simulink model "QCar2_DetailedScenario-2025a"  (R2025a)
settings: Solver=ode2  StartTime=0.0  StopTime=inf  FixedStep=1/100  RelTol=1e-3  EnableMultiTasking=on
model workspace (MAT data in the model file):
  XY_OFFSET = Simulink.Parameter
  XY_OFFSET.Value = [0 0]
  XY_OFFSET.Complexity = 'real'
  XY_OFFSET.Dimensions = [1 2]
  XY_OFFSET.DataType = 'double'
  camera_rate = Simulink.Parameter
  camera_rate.Value = Simulink.data.Expression
  camera_rate.Value.ExpressionString = "qc_get_step_size * ceil(1/30 / qc_get_step_size)"
  camera_rate.Complexity = 'real'
  camera_rate.Dimensions = -1
  camera_rate.DataType = 'auto'
  depth_rate = Simulink.Parameter
  depth_rate.Value = Simulink.data.Expression
  depth_rate.Value.ExpressionString = "qc_get_step_size * ceil(1/30 / qc_get_step_size)"
  depth_rate.Complexity = 'real'
  depth_rate.Dimensions = -1
  depth_rate.DataType = 'auto'
  path_to_pickup = Simulink.Parameter
  path_to_pickup.Value = [-12.05  -8.3; -10.5  -9; -8  -10; -6  -10.5; -4  -10.8; -2  -10.9; 0  -10.95; 2  -10.95; 4  -10.9; 6  -10.85; 8  -10.85; 10  -10.9; 12  -10.92; 14  -10.92; 16  -10.5; 18  -9; 19.5  -7.5; 20.5  -5.5; 21  -4; 21.5  -3; 21.8  -1.5; 22  0; 22.1  2; 22.15  4; 22.15  6; 22.15  8; 22.15  10; 22.15  12; 22.15  14; 22.15  16; 22.15  18; 22.1  20; 22.1  22; 22.1  24; 22.1  26; 22.1  28; 22.05  30; 22  32; 21.9  34; 21.7  36; 21.4  38; 21  40; 20.5  41.5; 19.8  43; 18.8  44; 17.5  44.5; 16  44.8; 14  44.9; 12  44.92; 10  44.92; 8  44.92; 6  44.92; 4  44.92; 2  44.92; 1.25  44.5; 1.25  43.95]
  path_to_pickup.Complexity = 'real'
  path_to_pickup.Dimensions = [56 2]
  path_to_pickup.DataType = 'double'
  path_to_pickup_tight = Simulink.Parameter
  path_to_pickup_tight.Value = [-12.05  -8.3; -10.5  -9; -8  -10; -6  -10.5; -4  -10.8; -2  -10.9; 0  -10.95; 2  -10.95; 4  -10.9; 6  -10.85; 8  -10.85; 10  -10.9; 12  -10.92; 14  -10.92; 16  -10.5; 18  -9; 19.5  -7.5; 20.5  -5.5; 21  -4; 21.5  -3; 21.8  -1.5; 22  0; 22.1  2; 22.15  4; 22.15  6; 22.15  8; 22.15  10; 22.15  12; 22.15  14; 22.15  16; 22.15  18; 22.1  20; 22.1  22; 22.1  24; 22.1  26; 22.1  28; 22.05  30; 22  32; 21.9  34; 21.7  36; 21.4  38; 21  40; 20.5  41.5; 19.8  43; 18.8  44; 17.5  44.5; 16  44.8; 14  44.9; 12  44.92; 10  44.92; 8  44.92; 6  44.92; 4  44.92; 2  44.92; 1.25  44.5; 1.25  43.95]
  path_to_pickup_tight.Complexity = 'real'
  path_to_pickup_tight.Dimensions = [56 2]
  path_to_pickup_tight.DataType = 'double'
undefined symbols (not defined in the file or in its folder): gcbh, HIL, JPEG, Point, qc_get_step_size, Video3D, video_display_show
libraries: quarc_library x37, simulink x16
(part 1 of 3)
settings Model: SimulationMode=external  ExtModeTrigDuration=10000  Creator=User  LastModifiedBy=ricar
settings SolverCC: PositivePriorityOrder=on  AutoInsertRateTranBlk=on
settings DataIOCC: ReturnWorkspaceOutputs=off
settings DebuggingCC: AlgebraicLoopMsg=none  ParameterPrecisionLossMsg=none  UnconnectedInputMsg=warning  UnconnectedOutputMsg=warning  UnconnectedLineMsg=warning  ArithmeticOperatorsInVariantConditions=warning
settings ModelReferenceCC: EnableRefExpFcnMdlSchedulingChecks=on
settings SFSimCC: SimUseLocalCustomCode=off  CustomCodeUndefinedFunction=UseInterfaceOnly
settings RTWCC: RTWUseLocalCustomCode=off  Toolchain=QUARC win64 | nmake (64-bit Windows)  BuildConfiguration=Faster Runs  GPUComputeCapability=3.5

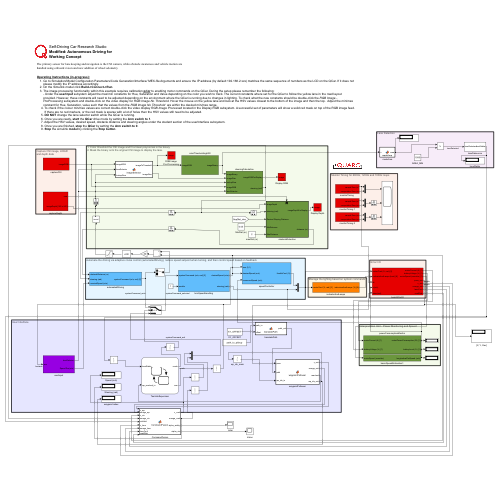
[thumbnail: Simulink's stored preview of the top-level diagram]
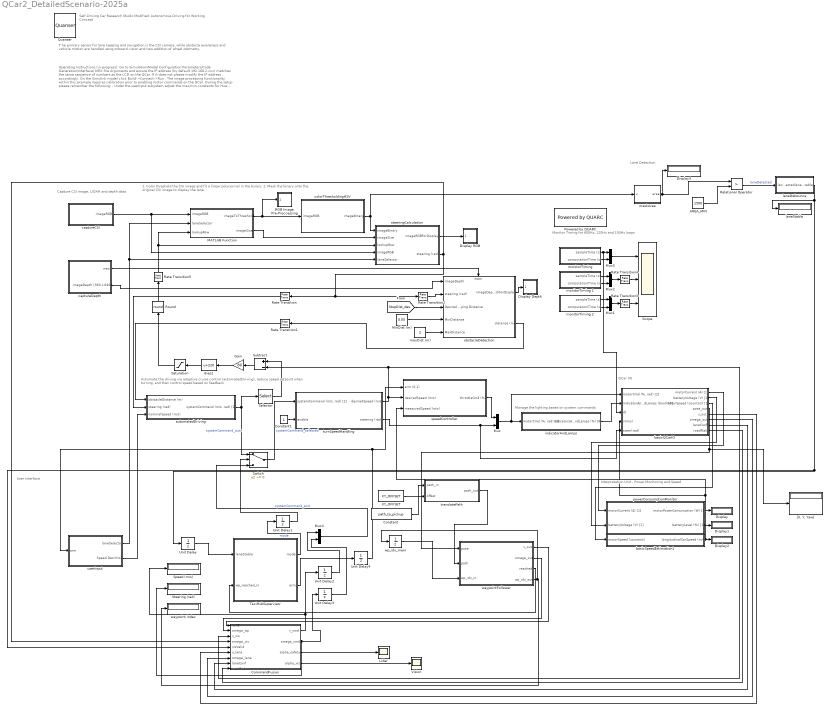
== system QCar2_DetailedScenario-2025a ==
  note: User Interface
  note: Operating Instructions (in-progress):
      | Go to Simulation/Model Configuration Parameters/Code Generation/Interface/ MEX-file Arguments and ensure the IP address (by default 192.168.2.xxx) matches the same sequence of numbers as the LCD on the QCar. If it does not please modify the IP address accordingly.
      | On the Simulink model click Build->Connect->Run .
      | The image processing functionality within this example requires calibration prior to enabling motor commands on the QCar. During the setup please remember the following:
      | - Under the userInput subystem adjust the max/min constants for Hue, Saturation and Value depending on the color you wish to track. The current constants where set for the QCar to follow the yellow lane in the road layout provided. However, these constants will need to be adjusted depending on the environment where the QCar is running due to changes in lighting. To check what the new constants should be double-click the RGB Image -PreProcessing subsystem and double-click on the video display for RGB Image No Threshold . Hover the mouse on the yellow lane and look at the HSV values closest to the bottom of the image and then the top. Adjust the min/max constant for Hue, Saturation, value such that the values from the RGB Image No Threshold are within the desired min/max range.
      | 4. To check if the colour min/max values are correct double-click the video display RGB Image Processed located in the Display RGB subsystem. A successful set of parameters will show a solid red mask on top of the RGB image feed.
      | If there are no red markers, or the red mask is sparse with a lot of holes then the HSV values still need to be adjusted.
      | 5. DO NOT change the lane selector switch while the QCar is running.
      | 6. Once you are ready, start the QCar drive mode by setting the Arm switch to 1 .
      | 7. Adjust the HSV values, desired speed, obstacle distance and steering angles under the student section of the userInterface subsystem.
      | 8. Once you are finished, stop the QCar by setting the Arm switch to 0 .
      | 9. Stop the simulink model by clicking the Stop button .
  note: Monitor Timing for 600Hz, 120Hz and 100Hz loops
  note: Manage the lighting based on system commands
  note: QCar I/O
  note: Automate the driving via adaptive cruise control (automatedDriving), reduce speed setpoint when turning, and then control speed based on feedback
  note: Self-Driving Car Research Studio
      | Modified: Autonomous Driving for Working Concept
  note: Capture CSI image, LIDAR
      | and depth data
  note: 1. Color threshold the CSI image and fit a linear polynomial in the binary.
      | 2. Mask the binary onto the original CSI image to display the lane.
  note: T he primary sensor for lane keeping and navigation is the CSI camera, while obstacle awareness and vehicle motion are handled using onboard vision and new addition of wheel odometry.
  note: Interpretation Unit - Power Monitoring and Speed
  note: Lane Detection
  AREA_MIN : Constant  Value=1500
  Bias1 : Bias  Bias=220  SaturateOnIntegerOverflow=off
  CommandFusion : MATLAB Function  TreatAsAtomicUnit=on
  Constant : Constant  Value=path_to_pickup
  Constant1 : Constant
  Display{,1..3} (4 alike) : Display
      Display settings: Decimation=0.5/qc_get_step_size
      Display1 settings: Decimation=0.5/qc_get_step_size
      Display2 settings: Decimation=0.5/qc_get_step_size
  Display Depth : Subsystem
  Display RGB : Subsystem
  Gain : Gain  Gain=80
  Lidar : Scope
      settings: ActiveDisplayYMinimum=0.063200000000000034  ActiveDisplayYMaximum=0.26320000000000005  DataLoggingVariableName=ScopeData6
  MATLAB Function : MATLAB Function  TreatAsAtomicUnit=on
  MinDist (m) : Constant  Value=0.05
  Mux{,1..4} (5 alike) : Mux  Inputs=2
  Powered by QUARC : quarc_library/Logos/Powered by QUARC
  Quanser : quarc_library/Logos/Quanser
  RGB Image Pre-Proccessing : Subsystem
  Rate Transition{,1,3..5} (5 alike) : RateTransition
  Rate Transition2 : RateTransition  Deterministic=off
  Relational Operator : RelationalOperator  Operator=>  OutDataTypeStr=boolean  RndMeth=Simplest  InputSameDT=off
  Round : Rounding  Operator=round
  Saturation : Saturate  UpperLimit=300  LowerLimit=220
  Scope : Scope  NumInputPorts=3
      settings: TimeSpan=60  Title=Timing: 500 Hz loop  ActiveDisplayYMinimum=-0.00084  ActiveDisplayYMaximum=0.00516  YLabel=s
  Selector : Selector  InputPortWidth=2  IndexOptions=Index vector (dialog)  Indices=[1]  OutputSizes=1
  Speed (m/s) : Display
  Steering (rad) : Display
  Subtract : Sum  Inputs=+-
  Switch : Switch  Criteria=u2 ~= 0  SaturateOnIntegerOverflow=off  InputSameDT=off
  "TaxiHubSupervisor " : Stateflow chart  TreatAsAtomicUnit=on
  Unit Delay{,1..4} (5 alike) : UnitDelay  SampleTime=-1  HasFrameUpgradeWarning=on
  Vision : Scope
      settings: ActiveDisplayYMinimum=-1  ActiveDisplayYMaximum=1  DataLoggingVariableName=ScopeData7
  XY_OFFSET : Constant  Value=XY_OFFSET
  "[X, Y, Yaw]" : Display
  automatedDriving : Subsystem
  basicQCarIO : Subsystem
  basicSpeedEstimation1 : Subsystem
  captureCSI : Subsystem
  captureDepth : Subsystem
  colorThresholdingHSV : Subsystem
  indicatorAndLamps : Subsystem
  laneDebounce : Subsystem
  laneStable : Display
  maskArea : MATLAB Function  TreatAsAtomicUnit=on
  maxDist (m) : Constant  Value=2
  "monitorTiming " : Subsystem
  monitorTiming 1 : Subsystem
  monitorTiming 2 : Subsystem
  obstacleDetection : Subsystem
  powerConsumptionMonitor : Subsystem
  speedController : Subsystem
  steeringCalculation : Subsystem
  translatePath : MATLAB Function  TreatAsAtomicUnit=on
  turnSpeedHandling : Subsystem
  userInput : Subsystem
  waypoint index : Display
  waypointFollower : MATLAB Function  TreatAsAtomicUnit=on
  wp_idx_mem : UnitDelay  InitialCondition=1  SampleTime=-1  HasFrameUpgradeWarning=on
  wires:
  Mux/1 -> basicQCarIO/1("motorCmd (%, rad) [2]"), indicatorAndLamps/1("motorCmd (%, rad) [2]")
  turnSpeedHandling/2(steering (rad)) -> basicQCarIO/5(steer(rad)), Mux/2
  Constant1/1 -> turnSpeedHandling/2(enable)
  indicatorAndLamps/1(indicatorsAndLamps (%) [8]) -> basicQCarIO/2(indicatorAndLamps (bool) [8])
  captureDepth/2(imageDepth [360 x 640]) -> obstacleDetection/1(imageDepth)
  obstacleDetection/2(distance (m)) -> Rate Transition1/1
  speedController/1(throttleCmd (%)) -> Mux/1
  Rate Transition/1 -> automatedDriving/2(steering (rad))
  Rate Transition1/1 -> automatedDriving/1(obstacleDistance (m))
  Rate Transition2/1 -> obstacleDetection/2(steering (rad))
  obstacleDetection/1(imageDepthForDisplay) -> Display Depth/1(Image)
  captureCSI/1(imageRGB) -> steeringCalculation/4(imageRGB), MATLAB Function/1(imageRGB)
  monitorTiming 2/2(computationTime (s)) -> Mux1/2
  monitorTiming 2/1(sampleTime (s)) -> Mux1/1
  monitorTiming 1/2(computationTime (s)) -> Mux2/2
  monitorTiming 1/1(sampleTime (s)) -> Mux2/1
  "monitorTiming "/2(computationTime (s)) -> Mux3/2
  "monitorTiming "/1(sampleTime (s)) -> basicQCarIO/3(dt), Mux3/1
  Mux2/1 -> Rate Transition4/1
  Mux1/1 -> Rate Transition3/1
  Mux3/1 -> Scope/1
  Rate Transition3/1 -> Scope/3
  Rate Transition4/1 -> Scope/2
  captureDepth/1(new) -> obstacleDetection/Enable
  steeringCalculation/2(steering (rad)) -> CommandFusion/4(omega_vis), Rate Transition2/1, Rate Transition/1
  colorThresholdingHSV/1(imageBinary) -> maskArea/1(u), steeringCalculation/1(imageBinary)
  steeringCalculation/1(imageRGBForDisplay) -> Display RGB/1(Image)
  MATLAB Function/1(imageToThreshold) -> RGB Image Pre-Proccessing/1(Image), colorThresholdingHSV/1(imageRGB)
  MATLAB Function/2(imageSize) -> steeringCalculation/2(imageSize)
  turnSpeedHandling/1(desiredSpeed (m/s)) -> speedController/2(desiredSpeed (m/s)), CommandFusion/3(v_vis), Subtract/2
  Gain/1 -> Bias1/1
  Saturation/1 -> Round/1
  Selector/1 -> Subtract/1
  Subtract/1 -> Gain/1
  Bias1/1 -> Saturation/1
  Rate Transition5/1 -> steeringCalculation/3(lookupRow), MATLAB Function/3(lookupRow)
  userInput/1(laneSelector) -> steeringCalculation/5(laneSelector), MATLAB Function/2(laneSelector)
  userInput/2(Speed Des(m/s)) -> automatedDriving/3(nominalSpeed (m/s))
  [StopDist_des] -> obstacleDetection/3(Desired Stoping Distance)
  maxDist (m)/1 -> obstacleDetection/5(MaxDistance)
  MinDist (m)/1 -> obstacleDetection/4(MinDistance)
  Round/1 -> Rate Transition5/1
  basicQCarIO/1(motorCurrent (A) [1]) -> powerConsumptionMonitor/1(motorCurrent (A) [1])
  basicQCarIO/2(batteryVoltage (V) [1]) -> powerConsumptionMonitor/2(batteryVoltage (V) [1])
  basicQCarIO/3(motorSpeed (counts/s) [1]) -> basicSpeedEstimation1/1(motorSpeed (counts/s))
  powerConsumptionMonitor/1(motorPowerConsumption (W) [1]) -> Display/1
  basicSpeedEstimation1/1(longitudinalCarSpeed (m/s)) -> basicQCarIO/4(v(m/s)), speedController/3(measuredSpeed (m/s)), Display2/1
  powerConsumptionMonitor/2(batteryLevel (%) [1]) -> Display1/1
  automatedDriving/1("systemCommand (m/s, rad) [2]") -> Selector/1, Switch/1  "systemCommand_auto"
  Mux4/1 -> Switch/3  "systemCommand_exit"
  Switch/1 -> turnSpeedHandling/1("systemCommand (m/s, rad) [2]")  "systemCommand_selected"
  maskArea/1(area) -> Display3/1, Relational Operator/1
  AREA_MIN/1 -> Relational Operator/2
  Relational Operator/1 -> laneDebounce/1(laneDetected)  "laneDetected"
  laneDebounce/1(laneStable) -> CommandFusion/5(visValid), Unit Delay/1, laneStable/1
  Unit Delay/1 -> "TaxiHubSupervisor "/1(laneStable)
  wp_idx_mem/1 -> waypointFollower/3(wp_idx_in)
  waypointFollower/4(wp_idx_out) -> waypoint index/1, wp_idx_mem/1
  waypointFollower/3(reached) -> "TaxiHubSupervisor "/2(wp_reached_in)
  "TaxiHubSupervisor "/1(mode) -> Unit Delay1/1  "mode"
  Unit Delay1/1 -> Switch/2
  Unit Delay2/1 -> Mux4/1
  "TaxiHubSupervisor "/2(arm) -> Unit Delay4/1
  Unit Delay4/1 -> userInput/1(arm), speedController/1(arm (0,1))
  Unit Delay3/1 -> Mux4/2
  XY_OFFSET/1 -> translatePath/2(offset)
  Constant/1 -> translatePath/1(path_in)
  translatePath/1(path_out) -> waypointFollower/2(path)
  basicQCarIO/4(pose_out) -> "[X, Y, Yaw]"/1, waypointFollower/1(pose)
  basicQCarIO/5(v_out) -> CommandFusion/6(v_lane)
  basicQCarIO/6(omega_out) -> CommandFusion/7(omega_lane)
  waypointFollower/1(v_out) -> CommandFusion/1(v_wp)
  CommandFusion/1(v_cmd) -> Speed (m/s)/1, Unit Delay2/1
  basicQCarIO/7(laneConf) -> CommandFusion/8(laneConf)
  basicQCarIO/8(roadRisk) -> CommandFusion/9(roadRisk)
  CommandFusion/3(alpha_safety) -> Lidar/1
  waypointFollower/2(omega_out) -> CommandFusion/2(omega_wp)
  CommandFusion/4(alpha_vis) -> Vision/1
  CommandFusion/2(omega_cmd) -> Steering (rad)/1, Unit Delay3/1

== system QCar2_DetailedScenario-2025a/Display Depth ==
  Image : Inport
  Channel : quarc_library/Signal Routing/Channel  channel=0  buffer_size=1
  Video Display : quarc_library/Multimedia/Video Display  Tag=QCar2_DetailedScenario/Display Depth/Video Display  sample_time=-1  use_hardware=on
  wires:
  Image/1 -> Channel/1
  Channel/1 -> Video Display/1

== system QCar2_DetailedScenario-2025a/Display RGB ==
  Image : Inport
  Channel : quarc_library/Signal Routing/Channel  channel=1  buffer_size=1
  Video Display : quarc_library/Multimedia/Video Display  Tag=QCar2_DetailedScenario/Display RGB/Video Display  sample_time=-1  use_hardware=on
  wires:
  Image/1 -> Channel/1
  Channel/1 -> Video Display/1

== system QCar2_DetailedScenario-2025a/RGB Image Pre-Proccessing ==
  Image : Inport
  Channel : quarc_library/Signal Routing/Channel  channel=2  buffer_size=1
  Video Display : quarc_library/Multimedia/Video Display  Tag="QCar2_DetailedScenario/RGB Image  Pre-Proccessing/Video Display"  sample_time=-1  use_hardware=on
  wires:
  Image/1 -> Channel/1
  Channel/1 -> Video Display/1

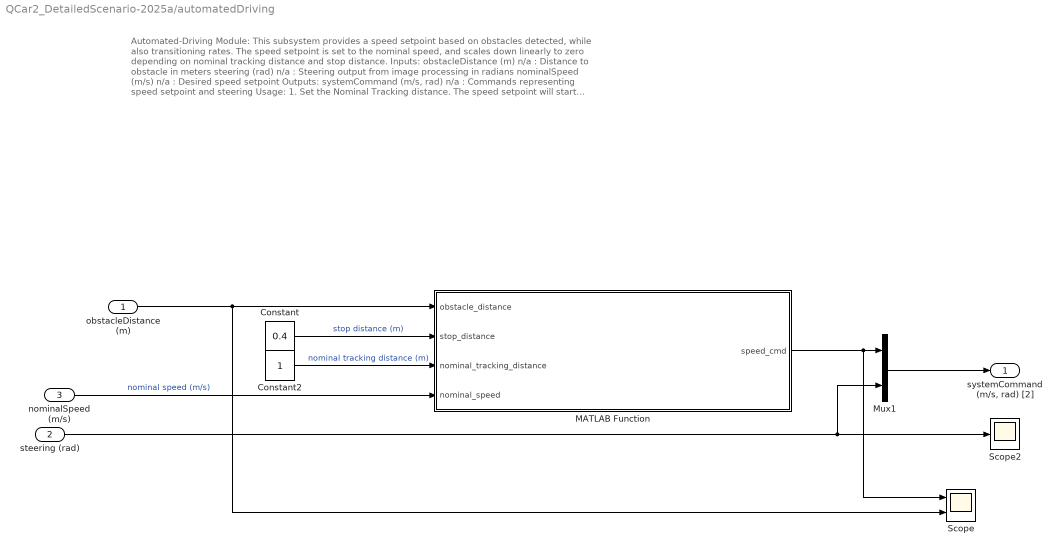
== system QCar2_DetailedScenario-2025a/automatedDriving ==
  note: Automated-Driving Module:
      |
      | This subsystem provides a speed setpoint based on obstacles detected, while also transitioning rates. The speed setpoint is set to the nominal speed, and scales down linearly to zero depending on nominal tracking distance and stop distance.
      |
      | Inputs:
      | obstacleDistance (m) n/a : Distance to obstacle in meters
      | steering (rad) n/a : Steering output from image processing in radians
      | nominalSpeed (m/s) n/a : Desired speed setpoint
      |
      | Outputs:
      | systemCommand (m/s, rad) n/a : Commands representing speed setpoint and steering
      |
      | Usage:
      | 1. Set the Nominal Tracking distance. The speed setpoint will start decreasing if the obstacle distance is less than this threshold.
      | 2. Set the Stop Distance. The speed setpoint will scale down to 0 when the the obstacle distance reaches this threshold.
  obstacleDistance (m) : Inport
  steering (rad) : Inport  Port=2
  nominalSpeed (m/s) : Inport  Port=3
  Constant : Constant  Value=0.4
  Constant2 : Constant
  MATLAB Function : MATLAB Function  TreatAsAtomicUnit=on
  Mux1 : Mux  Inputs=2
  Scope : Scope  NumInputPorts=2
      settings: ActiveDisplayYMinimum=-0.06597  ActiveDisplayYMaximum=1.21757
  Scope2 : Scope
      settings: ActiveDisplayYMinimum=-0.625  ActiveDisplayYMaximum=0.625  DataLoggingVariableName=ScopeData2
  "systemCommand (m/s, rad) [2]" : Outport  VectorParamsAs1DForOutWhenUnconnected=off
  wires:
  nominalSpeed (m/s)/1 -> MATLAB Function/4(nominal_speed)  "nominal speed (m/s)"
  Constant2/1 -> MATLAB Function/3(nominal_tracking_distance)  "nominal tracking distance (m)"
  Constant/1 -> MATLAB Function/2(stop_distance)  "stop distance (m)"
  MATLAB Function/1(speed_cmd) -> Scope/1, Mux1/1
  steering (rad)/1 -> Mux1/2, Scope2/1
  Mux1/1 -> "systemCommand (m/s, rad) [2]"/1
  obstacleDistance (m)/1 -> Scope/2, MATLAB Function/1(obstacle_distance)

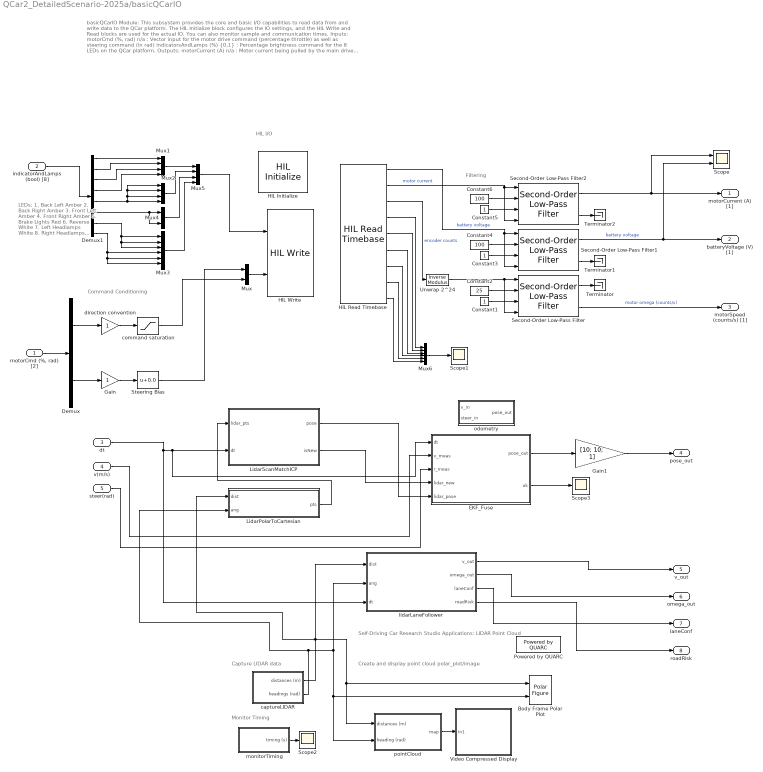
== system QCar2_DetailedScenario-2025a/basicQCarIO ==
  note: Filtering
  note: basicQCarIO Module:
      |
      | This subsystem provides the core and basic I/O capabilities to read data from and write data to the QCar platform. The HIL Initialize block configures the IO settings, and the HIL Write and Read blocks are used for the actual IO. You can also monitor sample and communication times.
      |
      | Inputs:
      | motorCmd (%, rad) n/a : Vector input for the motor drive command (percentage throttle) as well as steering command (in rad)
      | indicatorsAndLamps (%) {0,1} : Percentage brightness command for the 8 LEDs on the QCar platform.
      |
      | Outputs:
      | motorCurrent (A) n/a : Motor current being pulled by the main drive motor
      | batteryVoltage (V) {0, 12.6} : Current battery voltage reading
      | motorSpeed (counts/s) n/a : Drive motor speed measured using an encoder (do not confuse with wheel speed as this measurement is at the drive shaft)
  note: HIL I/O
  note: Command Conditioning
  note: LEDs:
      | 1. Back Left Amber
      | 2. Back Right Amber
      | 3. Front Left Amber
      | 4. Front Right Amber
      | 5. Brake Lights Red
      | 6. Reverse White
      | 7. Left Headlamps White
      | 8. Right Headlamps White
  note: Create and display point cloud polar_plot/image
  note: Self-Driving Car Research Studio
      | Applications: LIDAR Point Cloud
  note: Capture LIDAR data
  note: Monitor Timing
  "motorCmd (%, rad) [2]" : Inport
  indicatorAndLamps (bool) [8] : Inport  Port=2
  dt : Inport  Port=3
  v(m/s) : Inport  Port=4
  steer(rad) : Inport  Port=5
  Body Frame Polar Plot : quarc_library/Sinks/Figures/Polar Figure  figure_mode=Use figure window  figure_tag=figure1  axes_tag=axes1  plot_mode=Frame-based  minimum_rho=0  maximum_rho=5  minimum_theta=0  maximum_theta=360  zero_location=top  direction=counterclockwise  buffer_size=1000  update_rate=1  sample_time=-1  initial_position="898  139  994  602"  initial_visibility=off  line1_style=None  line1_width=0.5  line1_color=[0 0.4470 0.7410]  marker1=Point (.)  marker1_size=1  marker1_edge_color=[0 0.447059 0.741176]  marker1_face_color=[0 0.447059 0.741176]  line2_style=Solid line (-)  line2_width=0.5  line2_color=[0.85098 0.32549 0.0980392]  marker2=None  marker2_size=6  marker2_edge_color=[0.85098 0.32549 0.0980392]  marker2_face_color=[0.85098 0.32549 0.0980392]  line3_style=Solid line (-)  line3_width=0.5  line3_color=[0.929412 0.694118 0.12549]  marker3=None  marker3_size=6  marker3_edge_color=[0.929412 0.694118 0.12549]  marker3_face_color=[0.929412 0.694118 0.12549]  line4_style=Solid line (-)  line4_width=0.5  line4_color=[0.494118 0.184314 0.556863]  marker4=None  marker4_size=6  marker4_edge_color=[0.494118 0.184314 0.556863]  marker4_face_color=[0.494118 0.184314 0.556863]  line5_style=Solid line (-)  line5_width=0.5  line5_color=[0.466667 0.67451 0.188235]  marker5=None  marker5_size=6  marker5_edge_color=[0.466667 0.67451 0.188235]  marker5_face_color=[0.466667 0.67451 0.188235]
      settings: SourceProductName=QUARC Targets
  Constant1 : Constant
  Constant2 : Constant  Value=25
  Constant3 : Constant
  Constant4 : Constant  Value=100
  Constant5 : Constant
  Constant6 : Constant  Value=100
  Demux : Demux  Outputs=2
  Demux1 : Demux  Outputs=8
  EKF_Fuse : MATLAB Function  TreatAsAtomicUnit=on
  Gain : Gain
  Gain1 : Gain  Gain=[10; 10; 1]
  HIL Initialize : quarc_library/Data Acquisition/Generic/Configuration/HIL Initialize  object_name=HIL-1  board_type=qcar2  board_number=0@tcpip://localhost:18960  board_options=gyro_fs=250;gyro_rate=500;gyro_bw=125;gyro_ord=3;accel_fs=16;accel_rate=1000;accel_bw=250;accel_ord=3;temp_bw=4000;enc0_dir=0;enc1_dir=0;enc2_dir=0;steer_bias=0.05;  exclusive=off  active=on  hardware_clocks=[]  clock_modes=[]  initial_clock_frequencies=[]  set_clock_params_at_start=off  set_clock_params_at_switch_in=off  set_clock_frequencies_at_start=off  set_clock_frequencies_at_switch_in=off  analog_input_channels=[0:4]  analog_input_configurations=[]  analog_input_maximums=[3.3]  analog_input_minimums=[0]  set_analog_input_params_at_start=off  set_analog_input_params_at_switch_in=off  analog_output_channels=[]  analog_output_maximums=[]  analog_output_minimums=[]  initial_analog_outputs=[]  final_analog_outputs=[]  watchdog_analog_outputs=[]  set_analog_output_params_at_start=off  set_analog_output_params_at_switch_in=off  set_analog_outputs_at_start=off  set_analog_outputs_at_switch_in=off  set_analog_outputs_at_terminate=off  set_analog_outputs_at_switch_out=off  set_analog_outputs_on_watchdog=off  digital_input_channels=[0:14]  digital_output_channels=[11:26]  digital_output_configuration=[]  initial_digital_outputs=[0]  final_digital_outputs=[0]  watchdog_digital_outputs=[0]  set_digital_output_params_at_start=off  set_digital_output_params_at_switch_in=off  set_digital_outputs_at_start=on  set_digital_outputs_at_switch_in=off  set_digital_outputs_at_terminate=on  set_digital_outputs_at_switch_out=off  set_digital_outputs_on_watchdog=off  encoder_channels=[0:2]  quadrature=[4]  encoder_filter_frequency=100e6/1  initial_encoder_counts=[0]  set_encoder_params_at_start=on  set_encoder_params_at_switch_in=off  set_encoder_counts_at_start=on  set_encoder_counts_at_switch_in=off  pwm_channels=[0:1]  pwm_modes=[0]  pwm_frequency=180e6/4096  pwm_configuration=[0]  pwm_alignment=[0]  pwm_polarity=[1]  pwm_leading_deadband=[]  pwm_trailing_deadband=[]  initial_pwm_outputs=[0]  final_pwm_outputs=[0]  watchdog_pwm_outputs=[0]  set_pwm_params_at_start=on  set_pwm_params_at_switch_in=off  set_pwm_outputs_at_start=on  set_pwm_outputs_at_switch_in=off  set_pwm_outputs_at_terminate=on  set_pwm_outputs_at_switch_out=off  set_pwm_outputs_on_watchdog=off  other_output_channels=[1000 11000]  initial_other_outputs=[0]  final_other_outputs=[0]  watchdog_other_outputs=[0]  set_other_outputs_at_start=on  set_other_outputs_at_switch_in=off  set_other_outputs_at_terminate=on  set_other_outputs_at_switch_out=off  set_other_outputs_on_watchdog=off
  HIL Read Timebase : quarc_library/Data Acquisition/Generic/Timebases/HIL Read Timebase  object_name=HIL-1  clock=0  analog_channels=[2 4]  encoder_channels=[0]  digital_channels=[]  other_channels=[3000:3002 4000:4002]  active=on  vector_output=off  data_type_mode=Inherit via back propagation  encoder_data_type=double  digital_data_type=boolean  overflow_mode=Synchronize (for simulated cards only)  samples_in_buffer=max(ceil(1/qc_get_step_size), 1)*0+1
  HIL Write : quarc_library/Data Acquisition/Generic/Immediate I//O/HIL Write  object_name=HIL-1  analog_channels=[]  pwm_channels=[]  digital_channels=[17:18 25:26 11:16 19:24]  other_channels=[1000 11000]  sample_time=qc_get_step_size  active=on  vector_input=on
  LidarPolarToCartesian : MATLAB Function  TreatAsAtomicUnit=on
  LidarScanMatchICP : MATLAB Function  TreatAsAtomicUnit=on
  Mux : Mux  Inputs=2
  Mux1 : Mux
  Mux2 : Mux
  Mux3 : Mux  Inputs=6
  Mux4 : Mux  Inputs=2
  Mux5 : Mux
  Mux6 : Mux  Inputs=6
  Powered by QUARC : quarc_library/Logos/Powered by QUARC
  Scope : Scope  NumInputPorts=2
      settings: ActiveDisplayYMinimum=-1.03564  ActiveDisplayYMaximum=12.37845  DataLoggingVariableName=ScopeData4
  Scope1 : Scope
  Scope2 : Scope
      settings: ActiveDisplayYMinimum=-0.0098  ActiveDisplayYMaximum=0.1122
  Scope3 : Scope
      settings: ActiveDisplayYMinimum=-1  ActiveDisplayYMaximum=1  DataLoggingVariableName=ScopeData5
  Second-Order Low-Pass Filter : quarc_library/Continuous/Second-Order Low-Pass Filter  params_source=External (input ports)  input_width=1  input_zeta=1  input_init=0
  Second-Order Low-Pass Filter1 : quarc_library/Continuous/Second-Order Low-Pass Filter  params_source=External (input ports)  input_width=1  input_zeta=1  input_init=0
  Second-Order Low-Pass Filter2 : quarc_library/Continuous/Second-Order Low-Pass Filter  params_source=External (input ports)  input_width=1  input_zeta=1  input_init=0
  Steering Bias : Bias  Bias=0.0  SaturateOnIntegerOverflow=off
  Terminator : Terminator
  Terminator1 : Terminator
  Terminator2 : Terminator
  Unwrap 2^24 : quarc_library/Discontinuities/Inverse Modulus  modulus=16777215  output_derivative=off  output_revolutions=off  max_x=Inf  min_x=-Inf
  Video Compressed Display : Subsystem  LoadFcn=set_param(gcbh, 'UserData', gcb);  StartFcn=video_display_show([gcb, '/Video Display'], 'add', gcb);  mask(Video Compressed Display){algorithm=JPEG, quality=50, sample_time=-1, use_hardware=on}
      mask prompts: algorithm "Compression algorithm:"; quality "Compression quality (0-100):"; sample_time "Sample time (seconds):"; use_hardware "Use hardware acceleration for video display"
      mask help: Displays a video stream on the host, using compression to minimize bandwidth.
      mask init:
      | qc_set_display('Video\nCompressed\nDisplay');
      settings: UndoDeleteFcn=set_param(gcbh, 'UserData', gcb);  OpenFcn=video_display_show([gcb, '/Video Display'], 'show', gcb);  PreDeleteFcn=video_display_show([gcb, '/Video Display'], 'delete');
      settings: CopyFcn=|
      | set_param(gcbh, 'UserData', gcb);
      | set_param(gcbh, 'LinkStatus', 'none');
      settings: NameChangeFcn=|
      | video_display_show([get_param(gcbh, 'UserData'), '/Video Display'], 'rename', [gcb, '/Video Display']);
      | video_display_show([gcb, '/Video Display'], 'add', gcb);
      | set_param(gcbh, 'UserData', gcb);
      mask Help: web(qc_get_block_help_path(gcb));
      mask TypeOptions algorithm: Image Compress/algorithm
      mask TypeOptions quality: Image Compress/quality
      mask TypeOptions sample_time: Video Display/sample_time
      mask TypeOptions use_hardware: Video Display/use_hardware
      mask Display:
      | patch([0.98591 0.98591 0.62618 0.59072 0.56147   0.536   0.536  0.5441 0.56912 0.59207 0.60881 0.62276 0.63527 0.64364  0.6485  0.6485 0.64706 0.64499 0.63662 0.62411 0.61232 0.59837 0.58307 0.56147   0.536   0.536  0.5441  0.5747 0.60953 0.63662 0.67001  0.7034 0.72851 0.75425 0.77927 0.80294 0.82454 0.84119 0.85865 0.87395 0.88574 0.89339  0.8969 0.89969 0.89969 0.89267  0.8816 0.87044 0.85649  0.8384 0.81824 0.80294 0.78764 0.77513 0.76676 0.75776 0.76397 0.77513 0.79178 0.80987 0.82796 0.84326 0.86207 0.98528],[0.18689 0.05522 0.05522 0.05171 0.05171    0.05 0.18338 0.18338 0.19148 0.20435 0.22298 0.24863 0.28589 0.33125 0.38138 0.55139 0.59801 0.63761 0.68189 0.72149 0.74939 0.76694 0.77855 0.79367 0.79952 0.92768 0.92768 0.92768 0.92417 0.92066 0.91364  0.9032 0.89384 0.88106 0.86594 0.85073 0.82634 0.80537 0.77855 0.74363 0.70403 0.65858 0.61079 0.59099 0.41513 0.37202 0.31847 0.29048 0.25556 0.23342  0.2102 0.19382 0.18221 0.17285 0.16943 0.16124  0.1589 0.16241 0.16709 0.17168  0.1787 0.18221 0.18689 0.18689],[0.9,0.90,0.91])
      | patch([0.536 0.52601 0.46823 0.44528 0.41603 0.39101 0.35555 0.33116 0.31451 0.29291  0.2804 0.26717 0.25322 0.23999 0.22406 0.20732 0.19337 0.17528 0.15935 0.14396 0.13217 0.11759 0.10922 0.10085 0.09671 0.09392 0.09041 0.08906 0.08906 0.09464  0.0995 0.10778 0.11894 0.13145 0.14675 0.16349 0.17672 0.19409 0.20732 0.22406 0.23999 0.26159 0.27833 0.29849 0.31793 0.33602 0.35411 0.37085 0.39245 0.41603   0.536   0.536 0.53159 0.46409   0.446 0.42026 0.39587 0.37571 0.36113 0.34925 0.34088 0.33809 0.33809 0.34088 0.34583 0.35627 0.36392 0.38129 0.39587 0.41117 0.42719 0.44672  0.4676 0.48353 0.48353 0.52394   0.536],[0.05 0.04829 0.04712 0.04712 0.04829 0.05063 0.05405 0.05873 0.06107 0.06692 0.07043 0.07619 0.08087 0.08672 0.09482 0.10652 0.11696 0.13325  0.1508 0.17168 0.19499 0.22415 0.25439 0.28472 0.31379 0.35456 0.38489 0.41513 0.58055 0.63878 0.68774 0.72149 0.75641 0.78089 0.80537 0.82859 0.84029 0.85658 0.86594 0.87404  0.8834 0.89267 0.90086 0.90788 0.91247 0.91832 0.92066   0.923 0.92651 0.92768 0.92768 0.79952 0.79952 0.79952 0.79718 0.78899 0.77153 0.75056 0.72149 0.68072 0.62249  0.5549 0.41396 0.37085 0.33242 0.28121 0.25205 0.22181 0.20552 0.19499 0.18572 0.18221 0.17753 0.17636 0.17753  0.1787  0.1787],[0.9,0.90,0.91])
      | disp('Video\nCompressed\nDisplay');
  captureLIDAR : Subsystem
  command saturation : Saturate  UpperLimit=0.20  LowerLimit=-0.20
  direction convention : Gain
  lidarLaneFollower : MATLAB Function  TreatAsAtomicUnit=on
  "monitorTiming " : Subsystem
  odometry : Subsystem
  pointCloud : Subsystem
  motorCurrent (A) [1] : Outport  VectorParamsAs1DForOutWhenUnconnected=off
  batteryVoltage (V) [1] : Outport  Port=2  VectorParamsAs1DForOutWhenUnconnected=off
  motorSpeed (counts/s) [1] : Outport  Port=3  VectorParamsAs1DForOutWhenUnconnected=off
  pose_out : Outport  Port=4
  v_out : Outport  Port=5  OutDataTypeStr=double  PortDimensions=1
  omega_out : Outport  Port=6  OutDataTypeStr=double  PortDimensions=1
  laneConf : Outport  Port=7
  roadRisk : Outport  Port=8
  wires:
  Second-Order Low-Pass Filter2/1 -> Scope/1, motorCurrent (A) [1]/1
  Constant2/1 -> Second-Order Low-Pass Filter/2
  Unwrap 2^24/1 -> Second-Order Low-Pass Filter/1, Second-Order Low-Pass Filter/4
  Second-Order Low-Pass Filter/1 -> Terminator/1
  Constant3/1 -> Second-Order Low-Pass Filter1/3
  Second-Order Low-Pass Filter1/1 -> Scope/2, batteryVoltage (V) [1]/1  "battery voltage"
  Constant5/1 -> Second-Order Low-Pass Filter2/3
  Second-Order Low-Pass Filter1/2 -> Terminator1/1
  HIL Read Timebase/1 -> Second-Order Low-Pass Filter1/4, Second-Order Low-Pass Filter1/1  "battery voltage"
  Constant6/1 -> Second-Order Low-Pass Filter2/2
  Second-Order Low-Pass Filter/2 -> motorSpeed (counts/s) [1]/1  "motor omega (counts/s)"
  Second-Order Low-Pass Filter2/2 -> Terminator2/1
  Constant4/1 -> Second-Order Low-Pass Filter1/2
  Constant1/1 -> Second-Order Low-Pass Filter/3
  HIL Read Timebase/3 -> Unwrap 2^24/1  "encoder counts"
  HIL Read Timebase/2 -> Second-Order Low-Pass Filter2/1, Second-Order Low-Pass Filter2/4  "motor current"
  Mux5/1 -> HIL Write/1
  "motorCmd (%, rad) [2]"/1 -> Demux/1
  Mux3/1 -> Mux5/4
  Demux1/4 -> Mux1/4
  Demux1/3 -> Mux1/3
  Demux1/6 -> Mux4/2, Mux4/1
  Steering Bias/1 -> Mux/1
  Demux1/8 -> Mux3/5, Mux3/6, Mux3/4
  Mux1/1 -> Mux5/1
  Demux1/7 -> Mux3/2, Mux3/3, Mux3/1
  Demux/1 -> direction convention/1
  Demux1/5 -> Mux2/4, Mux2/3, Mux2/2, Mux2/1
  Mux2/1 -> Mux5/2
  Mux/1 -> HIL Write/2
  indicatorAndLamps (bool) [8]/1 -> Demux1/1
  Demux/2 -> Gain/1
  Mux4/1 -> Mux5/3
  command saturation/1 -> Mux/2
  Demux1/2 -> Mux1/2
  direction convention/1 -> command saturation/1
  Gain/1 -> Steering Bias/1
  Demux1/1 -> Mux1/1
  Mux6/1 -> Scope1/1
  HIL Read Timebase/9 -> Mux6/6
  HIL Read Timebase/7 -> Mux6/4
  HIL Read Timebase/5 -> Mux6/2
  HIL Read Timebase/8 -> Mux6/5
  HIL Read Timebase/6 -> Mux6/3
  HIL Read Timebase/4 -> Mux6/1
  "monitorTiming "/1(timing (s)) -> Scope2/1
  captureLIDAR/2(headings (rad)) -> LidarPolarToCartesian/2(ang), lidarLaneFollower/2(ang), Body Frame Polar Plot/2, pointCloud/2(heading (rad))
  pointCloud/1(map) -> Video Compressed Display/1(In1)
  captureLIDAR/1(distances (m)) -> lidarLaneFollower/1(dist), LidarPolarToCartesian/1(dist), pointCloud/1(distances (m)), Body Frame Polar Plot/1
  LidarPolarToCartesian/1(pts) -> LidarScanMatchICP/1(lidar_pts)
  LidarScanMatchICP/1(pose) -> EKF_Fuse/5(lidar_pose)
  LidarScanMatchICP/2(isNew) -> EKF_Fuse/4(lidar_new)
  dt/1 -> lidarLaneFollower/3(dt), EKF_Fuse/1(dt), LidarScanMatchICP/2(dt)
  v(m/s)/1 -> EKF_Fuse/2(v_meas)
  steer(rad)/1 -> EKF_Fuse/3(r_meas)
  EKF_Fuse/2(ok) -> Scope3/1
  EKF_Fuse/1(pose_out) -> Gain1/1
  Gain1/1 -> pose_out/1
  lidarLaneFollower/1(v_out) -> v_out/1
  lidarLaneFollower/2(omega_out) -> omega_out/1
  lidarLaneFollower/3(laneConf) -> laneConf/1
  lidarLaneFollower/4(roadRisk) -> roadRisk/1

== system QCar2_DetailedScenario-2025a/basicSpeedEstimation1 ==
  note: speedEstimation Module:
      |
      | This subsystem converts the motor speed measurements in counts/s to a useful longitudinal car speed in m/s.
      |
      | Inputs:
      | motorSpeed (counts/s) n/a : Drive motor speed measured using an encoder
      |
      | Outputs:
      | longitudinalCarSpeed (m/s) n/a : The platform's longitudinal speed (along the front-rear axis direction)
  note: (Diff. pinion*pinion)/(Spur*Diff. spur)
  note: v = 2*pi*r * omega (if omega is in rot/s)
      | v = r * omega (if omega is in rad/s)
      | r = 0.0342 m
  note: Estimate car speed from motor encoder counts rate
  motorSpeed (counts/s) : Inport
  counts to rotations : Gain  Gain=1/720/4
  gear ratios : Gain  Gain=(13*19)/(70*37)
  rot/s to rad/s : Gain  Gain=2*pi
  wheel radius : Gain  Gain=0.0342
  longitudinalCarSpeed (m/s) : Outport  VectorParamsAs1DForOutWhenUnconnected=off
  wires:
  gear ratios/1 -> rot/s to rad/s/1  "shaft speed (rots/s)"
  wheel radius/1 -> longitudinalCarSpeed (m/s)/1  "wheel speed (m/s)"
  counts to rotations/1 -> gear ratios/1  "motor speed (rot/s)"
  rot/s to rad/s/1 -> wheel radius/1  "wheel speed (rad/s)"
  motorSpeed (counts/s)/1 -> counts to rotations/1

== system QCar2_DetailedScenario-2025a/captureCSI ==
  note: Capture CSI RGB Information at 30 fps, 820 x 410
  note: captureCSI Module:
      |
      | This subsystem outputs the RGB Image captured from the associated CSI device
      |
      | Outputs:
      | RGB (uint8) : RGB Image [height, width, 3]
      | new (bool) : Boolean flag that is high (1) when the data is new
      |
      | Usage:
      | Double-click the Video Capture block and set the 'Device Identifier' parameter to the desired value.
      | Also set the desired resolution and frame rate.
      |
      | Sample Rate:
      | The sample rate for this model is defined as the model workspace variable camera_rate found under the Model Explorer/Model Workspace . For this subsystem the image acquisition is done at a rate of 30 Hz.
  Scope : Scope
      settings: ActiveDisplayYMinimum=-0.125  ActiveDisplayYMaximum=1.125  DataLoggingVariableName=ScopeData3
  Video Capture : quarc_library/Multimedia/Video Capture  source=device  device=3@tcpip://localhost:18964  filename=sample_movie.mov  value=[0 0; 0 0]  resolution=820 x 410  width=820  height=410  output_format=MATLAB RGB (HxWx3)  data_type=uint8  sample_time=camera_rate  brightness_override=Do not override  brightness=50.0  contrast_override=Do not override  contrast=50.0  hue_override=Do not override  hue=50.0  saturation_override=Do not override  saturation=50.0  sharpness_override=Do not override  sharpness=50.0  gamma_override=Do not override  gamma=50.0  coloreffect_override=Do not override  coloreffect=None  whitebalance_override=Do not override  whitebalance=50.0  backlightcompensation_override=Do not override  backlightcompensation=0.0  gain_override=Do not override  gain=50.0  pan_override=Do not override  pan=50.0  tilt_override=Do not override  tilt=50.0  roll_override=Do not override  roll=50.0  zoom_override=Do not override  zoom=0.0  exposure_override=Do not override  exposure=50.0  iris_override=Do not override  iris=50.0  mirror_override=Do not override  mirror=None  focus_override=Do not override  focus=0.0
      settings: SourceProductName=QUARC Targets
  imageRGB : Outport  VectorParamsAs1DForOutWhenUnconnected=off
  wires:
  Video Capture/1 -> imageRGB/1
  Video Capture/2 -> Scope/1

== system QCar2_DetailedScenario-2025a/captureDepth ==
  note: Depth Capture Module:
      |
      | This subsystem outputs the RGB and Depth Images captured from the Intel Realsense device
      |
      | Outputs:
      | Depth Data (m) : Depth Data [height, width]
      | Depth New? (bool) : Boolean flag that is high (1) when the data is new
      |
      | Usage:
      | Connect the New? ports to the Enable/Trigger port of Enabled/Triggered subsystems that contain your code when using the image data.
      |
      | Sample Rate:
      | The sample rate for this model is defined as the model workspace variable depth_rate found under the Model Explorer/Model Workspace . For this subsystem the image acquisition is done at a rate of 100 Hz.
  note: Capture Realsense Depth Information at 30 fps, 640 x 480
  Depth : quarc_library/Multimedia/Video3D Capture  object_name=Video3D-1  stream_type=Depth  stream_index=0  resolution=640 x 480  width=640  height=480  output_format=Distance in meters (HxW)  data_type=single  sample_time=depth_rate  camera_intrinsics=off  depth_scale=off  brightness_override=Do not override  brightness=50.0  contrast_override=Do not override  contrast=50.0  hue_override=Do not override  hue=50.0  saturation_override=Do not override  saturation=50.0  sharpness_override=Do not override  sharpness=50.0  gamma_override=Do not override  gamma=50.0  gain_override=Do not override  gain=50.0  backlightcompensation_override=Do not override  backlightcompensation=50.0  whitebalance_override=Automatic white balance  whitebalance=50.0  exposure_override=Automatic exposure  exposure=30.0  emitter=Enable laser emitter  preset=Do not set camera presets
  Terminator2 : Terminator
  Terminator3 : Terminator
  Terminator4 : Terminator
  Video3D Initialize : quarc_library/Multimedia/Video3D Initialize  object_name=Video3D-1  source=Device  identifier=0@tcpip://localhost:18965  file=sample.bag  sample_time=depth_rate  active=on
  new : Outport  VectorParamsAs1DForOutWhenUnconnected=off
  imageDepth [360 x 640] : Outport  Port=2  VectorParamsAs1DForOutWhenUnconnected=off
  wires:
  Depth/4 -> new/1
  Depth/1 -> imageDepth [360 x 640]/1
  Video3D Initialize/1 -> Terminator4/1
  Depth/3 -> Terminator3/1
  Depth/2 -> Terminator2/1

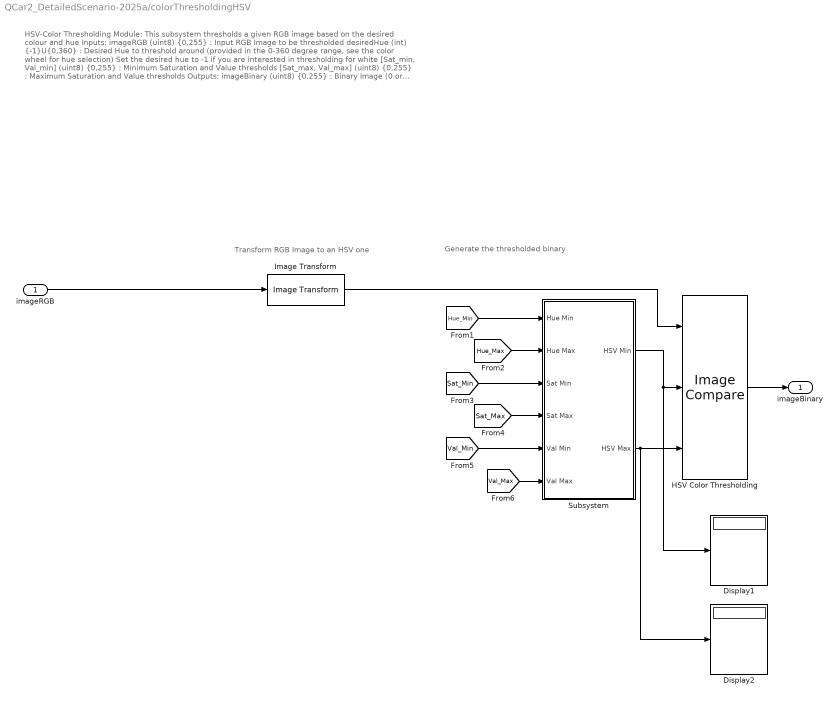
== system QCar2_DetailedScenario-2025a/colorThresholdingHSV ==
  note: HSV-Color Thresholding Module:
      |
      | This subsystem thresholds a given RGB image based on the desired colour and hue
      |
      | Inputs:
      | imageRGB (uint8) {0,255} : Input RGB Image to be thresholded
      | desiredHue (int) {-1}U{0,360} : Desired Hue to threshold around (provided in the 0-360 degree range, see the color wheel for hue selection)
      | Set the desired hue to -1 if you are interested in thresholding for white
      | [Sat_min, Val_min] (uint8) {0,255} : Minimum Saturation and Value thresholds
      | [Sat_max, Val_max] (uint8) {0,255} : Maximum Saturation and Value thresholds
      |
      | Outputs:
      | imageBinary (uint8) {0,255} : Binary Image (0 or 255 and no other value) representing the thresholding output
      |
      | Usage:
      | This module can be used when you are interested in thresholding for a certain hue regardless of the luminance. Compared to RGB thresholding which does not work well when the lighting conditions vary, HSV thresholding will correctly threshold for a hue (color) and allow you to specify a broad range of illuminance via the saturation and value thresholds. To broaden the range of hues accepted in the thresholding block, increase the Hue Threshold parameter.
  note: Transform RGB Image to an HSV one
  note: Generate the thresholded binary
  imageRGB : Inport
  Display1 : Display
  Display2 : Display
  HSV Color Thresholding : quarc_library/Image Processing/Generic/Image Compare  output_type=Combined (one HxW output)  source=External input ports  r_comparison=min <= pixel and pixel <= max with wrapping  r_minimum=30  r_maximum=70  g_comparison=min <= pixel and pixel <= max  g_minimum=60  g_maximum=100  b_comparison=min <= pixel and pixel <= max  b_minimum=40  b_maximum=80
      settings: SourceProductName=QUARC Targets
  Image Transform : quarc_library/Image Processing/Generic/Image Transform  algorithm=RGB to HSV  color_theme=KRYGCBMW  min_pixel=0  max_pixel=4000  contour_depth=1  focal_length=308  principal_point=[334 262]  radial_coeffs=[-0.3129 0.0907]  tangential_coeffs=[]  extrapolated_pixel=0  interpolation=nearest  row_coords=0  column_coords=0  output_height=480  output_width=640  angle=0  origin=[320 240]  output_origin=[320 240]  output_data_type=uint8
      settings: AttributesFormatString=(%<algorithm>)  SourceProductName=QUARC Targets
  Subsystem : Subsystem
  imageBinary : Outport  VectorParamsAs1DForOutWhenUnconnected=off
  wires:
  Image Transform/1 -> HSV Color Thresholding/1
  imageRGB/1 -> Image Transform/1
  [Hue_Max] -> Subsystem/2(Hue Max)
  [Val_Min] -> Subsystem/5(Val Min)
  [Hue_Min] -> Subsystem/1(Hue Min)
  [Sat_Min] -> Subsystem/3(Sat Min)
  [Sat_Max] -> Subsystem/4(Sat Max)
  [Val_Max] -> Subsystem/6(Val Max)
  Subsystem/2(HSV Max) -> HSV Color Thresholding/3, Display2/1
  Subsystem/1(HSV Min) -> Display1/1, HSV Color Thresholding/2
  HSV Color Thresholding/1 -> imageBinary/1

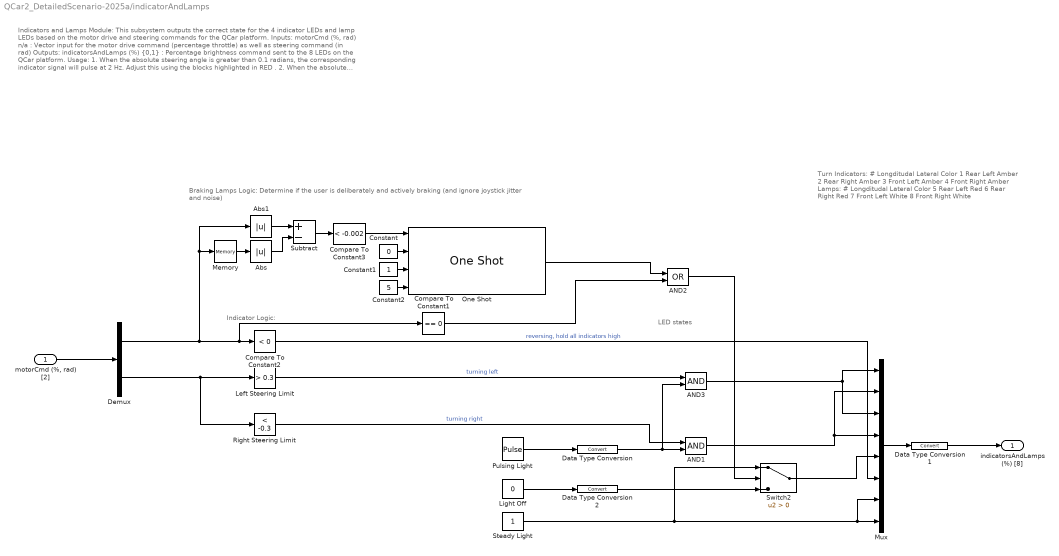
== system QCar2_DetailedScenario-2025a/indicatorAndLamps ==
  note: Indicators and Lamps Module:
      |
      | This subsystem outputs the correct state for the 4 indicator LEDs and lamp LEDs based on the motor drive and steering commands for the QCar platform.
      |
      | Inputs:
      | motorCmd (%, rad) n/a : Vector input for the motor drive command (percentage throttle) as well as steering command (in rad)
      |
      | Outputs:
      | indicatorsAndLamps (%) {0,1} : Percentage brightness command sent to the 8 LEDs on the QCar platform.
      |
      | Usage:
      | 1. When the absolute steering angle is greater than 0.1 radians, the corresponding indicator signal will pulse at 2 Hz. Adjust this using the blocks highlighted in RED .
      | 2. When the absolute motor drive command approaches 0, the brake lamps will receive 100% brightness command, and 0% brightness otherwise. Adjust this using the blocks highlighted in GREEN .
  note: Braking Lamps Logic:
      | Determine if the user is deliberately and actively braking (and ignore joystick jitter and noise)
  note: LED states
  note: Turn Indicators:
      | # Longditudal Lateral Color
      | 1 Rear Left Amber
      | 2 Rear Right Amber
      | 3 Front Left Amber
      | 4 Front Right Amber
      |
      | Lamps:
      | # Longditudal Lateral Color
      | 5 Rear Left Red
      | 6 Rear Right Red
      | 7 Front Left White
      | 8 Front Right White
  note: Indicator Logic:
  "motorCmd (%, rad) [2]" : Inport
  AND1 : Logic  IconShape=distinctive  AllPortsSameDT=off  OutDataTypeStr=boolean
  AND2 : Logic  Operator=OR  IconShape=distinctive  AllPortsSameDT=off  OutDataTypeStr=boolean
  AND3 : Logic  IconShape=distinctive  AllPortsSameDT=off  OutDataTypeStr=boolean
  Abs : Abs  SaturateOnIntegerOverflow=off
  Abs1 : Abs  SaturateOnIntegerOverflow=off
  Compare To Constant1 : simulink/Logic and Bit Operations/Compare To Constant  relop===  const=0  OutDataTypeStr=uint8
  Compare To Constant2 : simulink/Logic and Bit Operations/Compare To Constant  relop=<  const=0  OutDataTypeStr=boolean
  Compare To Constant3 : simulink/Logic and Bit Operations/Compare To Constant  relop=<  const=-0.002  OutDataTypeStr=boolean
  Constant : Constant  Value=0
  Constant1 : Constant
  Constant2 : Constant  Value=5
  Data Type Conversion : DataTypeConversion  SaturateOnIntegerOverflow=off  RndMeth=Floor
  Data Type Conversion1 : DataTypeConversion  SaturateOnIntegerOverflow=off  RndMeth=Floor
  Data Type Conversion2 : DataTypeConversion  SaturateOnIntegerOverflow=off  RndMeth=Floor
  Demux : Demux  Outputs=2
  Left Steering Limit : simulink/Logic and Bit Operations/Compare To Constant  relop=>  const=0.3  OutDataTypeStr=boolean
  Light Off : Constant  Value=0  OutDataTypeStr=boolean
  Memory : Memory
  Mux : Mux  Inputs=8
  One Shot : quarc_library/Discontinuities/One Shot  trigger_type=Falling edge  redun_pulse=Ignore extraneous pulse  width_source=External input port  pulse_width=100
      settings: SourceProductName=QUARC Targets
  Pulsing Light : DiscretePulseGenerator  Period=0.5/qc_get_step_size  PulseWidth=0.5/2/qc_get_step_size  SampleTime=qc_get_step_size
  Right Steering Limit : simulink/Logic and Bit Operations/Compare To Constant  relop=<  const=-0.3  OutDataTypeStr=boolean
  Steady Light : Constant  OutDataTypeStr=boolean
  Subtract : Sum  Inputs=+-
  Switch2 : Switch  Criteria=u2 > Threshold  SaturateOnIntegerOverflow=off  InputSameDT=off
  indicatorsAndLamps (%) [8] : Outport  VectorParamsAs1DForOutWhenUnconnected=off
  wires:
  Data Type Conversion2/1 -> Switch2/3
  Demux/2 -> Right Steering Limit/1, Left Steering Limit/1
  Light Off/1 -> Data Type Conversion2/1
  One Shot/1 -> AND2/1
  Steady Light/1 -> Mux/7, Mux/8, Switch2/1
  Compare To Constant3/1 -> One Shot/1
  Constant2/1 -> One Shot/4
  Right Steering Limit/1 -> AND1/1  "turning right"
  Mux/1 -> Data Type Conversion1/1
  Constant/1 -> One Shot/2
  Pulsing Light/1 -> Data Type Conversion/1
  Abs/1 -> Subtract/2
  Memory/1 -> Abs/1
  Abs1/1 -> Subtract/1
  Data Type Conversion/1 -> AND3/2, AND1/2
  Data Type Conversion1/1 -> indicatorsAndLamps (%) [8]/1
  Left Steering Limit/1 -> AND3/1  "turning left"
  Switch2/1 -> Mux/5
  Constant1/1 -> One Shot/3
  Demux/1 -> Compare To Constant1/1, Compare To Constant2/1, Memory/1, Abs1/1
  AND3/1 -> Mux/1, Mux/3
  "motorCmd (%, rad) [2]"/1 -> Demux/1
  Subtract/1 -> Compare To Constant3/1
  AND1/1 -> Mux/2, Mux/4
  Compare To Constant2/1 -> Mux/6  "reversing, hold all indicators high"
  Compare To Constant1/1 -> AND2/2
  AND2/1 -> Switch2/2

== system QCar2_DetailedScenario-2025a/laneDebounce ==
  laneDetected : Inport
  Add : Sum
  N : Constant  Value=10
  ONE : Constant
  ZERO : Constant  Value=0
  countSwitch : Switch  Criteria=u2 ~= 0  SaturateOnIntegerOverflow=off  InputSameDT=off
  count_z : UnitDelay  SampleTime=-1  HasFrameUpgradeWarning=on
  geN : RelationalOperator  OutDataTypeStr=boolean  RndMeth=Simplest  InputSameDT=off
  satN : Saturate  UpperLimit=10  LowerLimit=0
  laneStable : Outport
  wires:
  count_z/1 -> Add/1
  ONE/1 -> Add/2
  Add/1 -> satN/1
  satN/1 -> countSwitch/1
  laneDetected/1 -> countSwitch/2
  ZERO/1 -> countSwitch/3
  countSwitch/1 -> geN/1, count_z/1
  N/1 -> geN/2
  geN/1 -> laneStable/1

== system QCar2_DetailedScenario-2025a/monitorTiming  ==
  note: moniorTiming Module:
      |
      | This subsystem outputs the sample time and computation time of the model.
      |
      | Outputs:
      | sampleTime (s) n/a : Sample time (unfiltered and filtered) in seconds.
      | computationTime (s) n/a : Computation time (unfiltered and filtered) in seconds.
      |
      | Usage:
      | Compare the Sample Time (s) output to a constant (qc_get_step_size) to monitor whether or not the desired sample time is being achieved. The Computation Time (s) values should be lower than the corresponding sample time value to ensure that the solver has enough time per time step.
  note: Timing Performance
  Computation Time : quarc_library/Sources/Time/Computation Time  sample_time=qc_get_step_size  use_model=on  use_cpu_time=off
  Constant : Constant  Value=qc_get_step_size  SampleTime=-1
  Mux : Mux  Inputs=2
  Sample Time : quarc_library/Sources/Time/Sample Time  Priority=-99  sample_time=qc_get_step_size
  sampleTime (s) : Outport  VectorParamsAs1DForOutWhenUnconnected=off
  computationTime (s) : Outport  Port=2  VectorParamsAs1DForOutWhenUnconnected=off
  wires:
  Computation Time/1 -> computationTime (s)/1
  Constant/1 -> Mux/2
  Sample Time/1 -> Mux/1
  Mux/1 -> sampleTime (s)/1

== system QCar2_DetailedScenario-2025a/monitorTiming 1 ==
  note: Timing Performance
  note: moniorTiming Module:
      |
      | This subsystem outputs the sample time and computation time of the model.
      |
      | Outputs:
      | sampleTime (s) n/a : Sample time (unfiltered and filtered) in seconds.
      | computationTime (s) n/a : Computation time (unfiltered and filtered) in seconds.
      |
      | Usage:
      | Compare the Sample Time (s) output to a constant (qc_get_step_size) to monitor whether or not the desired sample time is being achieved. The Computation Time (s) values should be lower than the corresponding sample time value to ensure that the solver has enough time per time step.
  Computation Time : quarc_library/Sources/Time/Computation Time  sample_time=camera_rate  use_model=on  use_cpu_time=off
  Constant : Constant  Value=camera_rate  SampleTime=camera_rate
  Mux : Mux  Inputs=2
  Sample Time : quarc_library/Sources/Time/Sample Time  Priority=-99  sample_time=camera_rate
  sampleTime (s) : Outport  VectorParamsAs1DForOutWhenUnconnected=off
  computationTime (s) : Outport  Port=2  VectorParamsAs1DForOutWhenUnconnected=off
  wires:
  Computation Time/1 -> computationTime (s)/1
  Mux/1 -> sampleTime (s)/1
  Sample Time/1 -> Mux/1
  Constant/1 -> Mux/2

== system QCar2_DetailedScenario-2025a/monitorTiming 2 ==
  note: moniorTiming Module:
      |
      | This subsystem outputs the sample time and computation time of the model.
      |
      | Outputs:
      | sampleTime (s) n/a : Sample time (unfiltered and filtered) in seconds.
      | computationTime (s) n/a : Computation time (unfiltered and filtered) in seconds.
      |
      | Usage:
      | Compare the Sample Time (s) output to a constant (qc_get_step_size) to monitor whether or not the desired sample time is being achieved. The Computation Time (s) values should be lower than the corresponding sample time value to ensure that the solver has enough time per time step.
  note: Timing Performance
  Computation Time : quarc_library/Sources/Time/Computation Time  sample_time=depth_rate  use_model=on  use_cpu_time=off
  Constant : Constant  Value=depth_rate  SampleTime=depth_rate
  Mux : Mux  Inputs=2
  Sample Time : quarc_library/Sources/Time/Sample Time  Priority=-99  sample_time=depth_rate
  sampleTime (s) : Outport  VectorParamsAs1DForOutWhenUnconnected=off
  computationTime (s) : Outport  Port=2  VectorParamsAs1DForOutWhenUnconnected=off
  wires:
  Constant/1 -> Mux/2
  Sample Time/1 -> Mux/1
  Mux/1 -> sampleTime (s)/1
  Computation Time/1 -> computationTime (s)/1
